simulink model "INP_KEY_test"  (R2024b)
settings: Solver=VariableStepAuto  StartTime=0.0  StopTime=10.0  RelTol=1e-3
libraries: simulink x1, INP_KEY x1
settings Model: Creator=blatak  LastModifiedBy=blatak

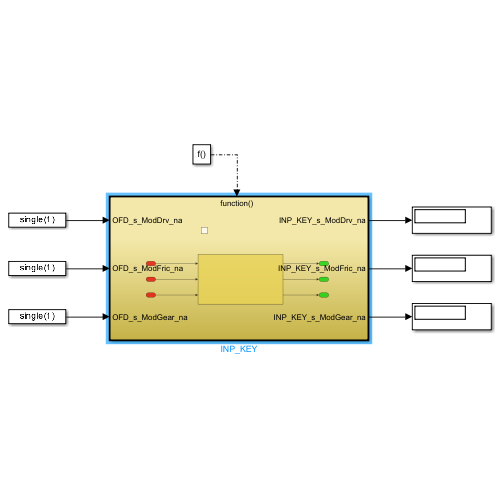
[thumbnail: Simulink's stored preview of the top-level diagram]
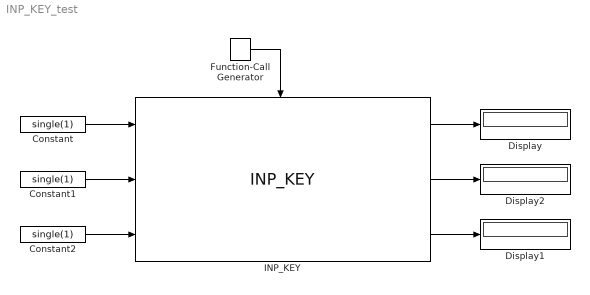
== system INP_KEY_test ==
  Constant : Constant  Value=single(1)
  Constant1 : Constant  Value=single(1)
  Constant2 : Constant  Value=single(1)
  Display : Display
  Display1 : Display
  Display2 : Display
  Function-Call Generator : simulink/Ports & Subsystems/Function-Call Generator  sample_time=0.005  numberOfIterations=1  DisallowWideOutput=off
  INP_KEY : INP_KEY/INP_KEY  SystemSampleTime=-1  VariantActivationTime=update diagram  AllowFlexibleInterface=on  Latency=0  AutoFrameSizeCalculation=off
  wires:
  Function-Call Generator/1 -> INP_KEY/Trigger
  Constant/1 -> INP_KEY/1
  Constant1/1 -> INP_KEY/2
  Constant2/1 -> INP_KEY/3
  INP_KEY/1 -> Display/1
  INP_KEY/2 -> Display2/1
  INP_KEY/3 -> Display1/1
